simulink model "Reaching_real"  (R2024b)
settings: Solver=FixedStepDiscrete  StartTime=0.0  StopTime=inf  FixedStep=0.001  RelTol=1e-3
libraries: PhanTorque_3Dof_Library_64Bits x1, vrlib x1
settings Model: Creator=carlos.aldana  LastModifiedBy=Wassim
settings SolverCC: AlgebraicLoopSolver=TrustRegion
settings DataIOCC: LimitDataPoints=on  SaveFormat=Array  ReturnWorkspaceOutputs=off
settings OptimizationCC: BlockReduction=off  BooleanDataType=off  LifeSpan=inf
settings DebuggingCC: SaveWithParameterizedLinksMsg=none  UnderspecifiedInitializationDetection=Classic  MergeDetectMultiDrivingBlocksExec=none  SignalResolutionControl=TryResolveAllWithWarning  UnconnectedInputMsg=warning  UnconnectedOutputMsg=warning  UnconnectedLineMsg=warning  AllowSymbolicDim=off  SFUnexpectedBacktrackingDiag=warning  SFNoUnconditionalDefaultTransitionDiag=warning  SFExecutionAtInitializationDiag=none  ArithmeticOperatorsInVariantConditions=warning
settings HardwareCC: ProdBitPerPointer=32  ProdBitPerSizeT=32  ProdBitPerPtrDiffT=32  ProdLargestAtomicFloat=None  ProdIntDivRoundTo=Undefined  ProdEndianess=Unspecified  ProdWordSize=32  ProdHWDeviceType=32-bit Generic  TargetUnknown=on
settings ModelReferenceCC: EnableRefExpFcnMdlSchedulingChecks=on  PropagateSignalLabelsOutOfModel=off
settings SFSimCC: SimUseLocalCustomCode=off  CustomCodeUndefinedFunction=UseInterfaceOnly
settings RTWCC: RTWUseLocalCustomCode=off  GPUComputeCapability=3.5  DLArmComputeVersion=19.05
settings CodeAppCC: StateflowObjectComments=on
settings GRTTargetCC: TargetLangStandard=C89/C90 (ANSI)
settings ConfigComp: CovMetricSettings=dw  CovSaveCumulativeToWorkspaceVar=on  CovSaveSingleToWorkspaceVar=on  CovExternalEMLEnable=off  CovSFcnEnable=off

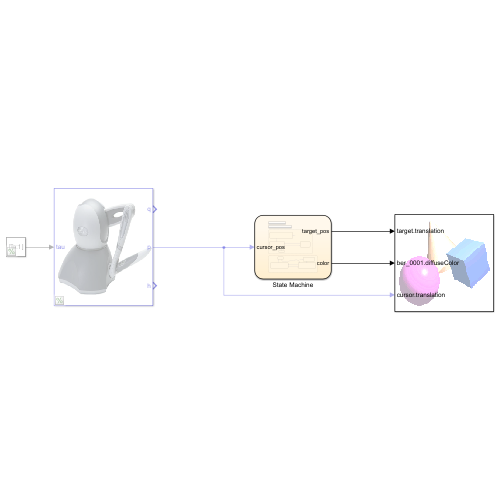
[thumbnail: Simulink's stored preview of the top-level diagram]
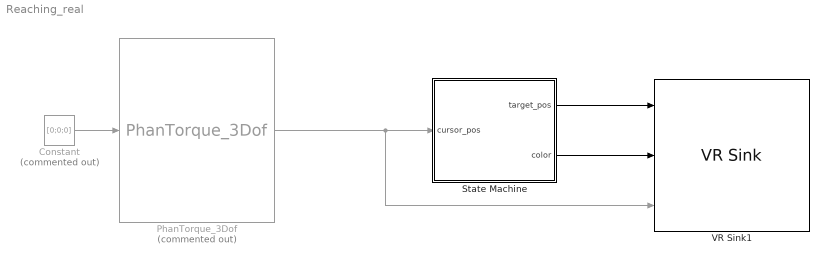
== system Reaching_real ==
  Constant : Constant  Commented=on  Value=[0;0;0]
  PhanTorque_3Dof : PhanTorque_3Dof_Library_64Bits/PhanTorque_3Dof  Commented=on  Haptic_Name='Default Device'
  State Machine : Stateflow chart  TreatAsAtomicUnit=on
  VR Sink1 : vrlib/VR Sink  InstantiateOnLoad=on  SampleTime=0.1  ViewEnable=on  RemoteChange=off  RemoteView=off  FieldsWritten=target.translation.3.1.1.double#ber_0001.diffuseColor.3.1.1.double#cursor.translation.3.1.1.double  WorldFileName=VR_centerAndTarget.wrl  AutoView=off  VideoDimensions=[]  AllowVariableSize=off
  wires:
  PhanTorque_3Dof/2 -> VR Sink1/3, State Machine/1(cursor_pos)
  State Machine/1(target_pos) -> VR Sink1/1
  State Machine/2(color) -> VR Sink1/2
  Constant/1 -> PhanTorque_3Dof/1

== stateflow chart Reaching_real/State Machine ==
  state TargetManager [parallel]
    settings: executionOrder=2
    state START
      entry:
      counter = 1;
      targets = generateTargets(radius, numTargets);
      randomTargets = generateRandomTargets(targets, numRepetitions);
    state ReachBoundaryTarget
      entry:
      target_pos = randomTargets(counter, : );
      holdTime = 1;
      exit:
      counter = counter + 1;
    state ReachCentralTarget
      entry:
      target_pos = [0,0,0];
      holdTime = 2;
    state FINISH
      end
    (default) -> START
    START -> ReachBoundaryTarget
    ReachCentralTarget -> ReachBoundaryTarget : [in(Feedback.TimerExpired)]{resetTimer = 1}
    ReachBoundaryTarget -> ReachCentralTarget [order 2] : [in(Feedback.TimerExpired)]{resetTimer = 1}
    ReachBoundaryTarget -> FINISH [order 1] : [counter>=numRepetitions]
  state Feedback [parallel]
    settings: executionOrder=1
    state TimerExpired
    state INIT
      entry:
      target_pos = [0,0,0];
      holdTime = 100; %Any high value
    state onTarget
      entry, during:
      distance = norm(cursor_pos(1:2) - target_pos(1:2));
      color = [0 1 0];
    state offTarget
      entry, during:
      distance = norm(cursor_pos(1:2) - target_pos(1:2));
      color = [1 0 0];
      resetTimer = 0;
    (default) -> INIT
    onTarget -> TimerExpired [order 2] : [after(holdTime, sec)]
    TimerExpired -> offTarget : [resetTimer == 1]
    INIT -> offTarget
    offTarget -> onTarget : [distance<=threshold]
    onTarget -> offTarget [order 1] : [distance>threshold]
  data: targets function_output; radius function_input; numTargets function_input; targets function_input; numRepetitions function_input; randomTargets function_output; target_pos output; counter local; cursor_pos input size=[1 3]; color output; baseNumbers local; extraNumbers local; i local; idx local; k local; numPoints local; numRepetitions constant double =10; randomNumbers local; randomTargets local size=[numRepetitions, 3]; targets local double size=[numTargets, 3]; theta local; x local; y local; threshold constant double =0.01; distance local; numTargets constant double =8; radius constant double =0.1; holdTime local; resetTimer local
  function targets = generateTargets(radius, numTargets):
    | function targets = generateTargets(radius, numTargets)
    |     targets = zeros(numTargets, 3);
    |     for k = 0:numTargets-1
    |         theta = 2 * pi * k / numTargets;
    |         x = radius * cos(theta);
    |         y = radius * sin(theta);
    |         targets(k+1, :) = [x, y, 0];
    |     end
    | end
  function randomTargets = generateRandomTargets(targets, numRepetitions):
    | function randomTargets = generateRandomTargets(targets, numRepetitions)
    |     numPoints = size(targets, 1); % Get the number of points
    |     % Generate the list of random numbers
    |     if numRepetitions <= numPoints
    |         % Non-repeating case
    |         randomNumbers = randperm(numPoints, numRepetitions);
    |     else
    |         % Repeating case: Ensure all numbers from 1 to numPoints are included at least once
    |         baseNumbers = randperm(numPoints); % Include 1 to numPoints at least once
    |         extraNumbers = randi(numPoints, 1, numRepetitions - numPoints); % Fill the rest with random numbers
    |         randomNumbers = [baseNumbers, extraNumbers];
    |     end
    |     % Preallocate the randomTargets matrix
    |     randomTargets = zeros(numRepetitions, 3);
    |     % Populate the randomTargets matrix
    |     for i = 1:numRepetitions
    |         idx = randomNumbers(i);         % Get the random index
    |         randomTargets(i, :) = targets(idx, :);
    |     end
    | end
